simulink model "SimpleDoubleMotorModel"  (R2024a)
settings: Solver=VariableStepAuto  StartTime=0.0  StopTime=10.0  RelTol=1e-3
values from neighbouring files (symbols this model uses):
  Ak = Ak_func(x0sk,u0k,z0k)    [Parameter.m]
  bk = bk_func(x0sk,u0k,z0k)    [Parameter.m]
  ck = ck_func(x0sk,u0k,z0k)    [Parameter.m]
settings Model: Creator=Jakob Reindl  LastModifiedBy=Jakob Reindl

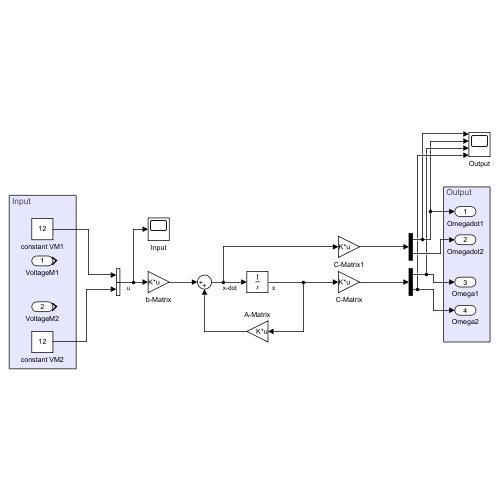
[thumbnail: Simulink's stored preview of the top-level diagram]
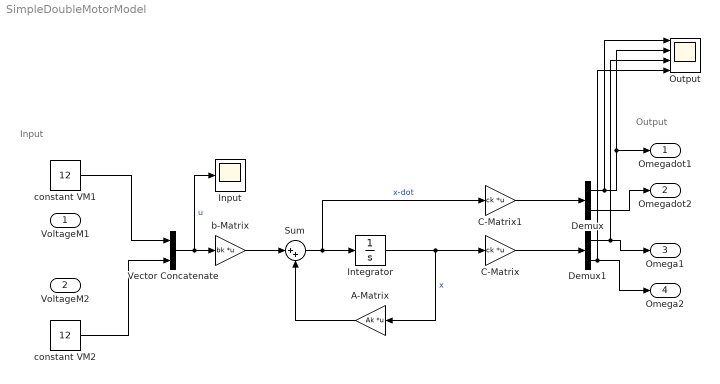
== system SimpleDoubleMotorModel ==
  note: Output
  note: Input
  VoltageM1 : Inport
  VoltageM2 : Inport  Port=2
  A-Matrix : Gain  Gain=Ak  Multiplication=Matrix(K*u)
  C-Matrix : Gain  Gain=ck  Multiplication=Matrix(K*u)
  C-Matrix1 : Gain  Gain=ck  Multiplication=Matrix(K*u)
  Demux : Demux  Outputs=2
  Demux1 : Demux  Outputs=2
  Input : Scope
  Integrator : Integrator
  Output : Scope  NumInputPorts=4
  Sum : Sum  Inputs=|++
  Vector Concatenate : Concatenate
  b-Matrix : Gain  Gain=bk  Multiplication=Matrix(K*u)
  constant VM1 : Constant  Value=12
  constant VM2 : Constant  Value=12
  Omegadot1 : Outport
  Omegadot2 : Outport  Port=2
  Omega1 : Outport  Port=3
  Omega2 : Outport  Port=4
  wires:
  C-Matrix1/1 -> Demux/1
  A-Matrix/1 -> Sum/2
  Vector Concatenate/1 -> Input/1, b-Matrix/1  "u"
  C-Matrix/1 -> Demux1/1
  Integrator/1 -> A-Matrix/1, C-Matrix/1  "x"
  Sum/1 -> C-Matrix1/1, Integrator/1  "x-dot"
  b-Matrix/1 -> Sum/1
  Demux/1 -> Output/1, Output/2, Omegadot1/1
  Demux/2 -> Omegadot2/1
  Demux1/1 -> Omega1/1, Output/3
  Demux1/2 -> Omega2/1, Output/4
  constant VM1/1 -> Vector Concatenate/1
  constant VM2/1 -> Vector Concatenate/2
